simulink subsystem "AddressToWordSelector"  (R2024b)
settings: Solver=VariableStepAuto  StartTime=0.0  StopTime=10.0  RelTol=1e-3
libraries: simulink x1
settings Model: Creator=stefano  LastModifiedBy=stefano

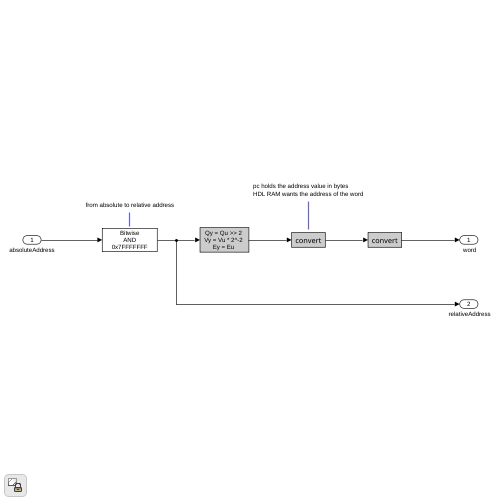
[thumbnail: Simulink's stored preview of the top-level diagram]
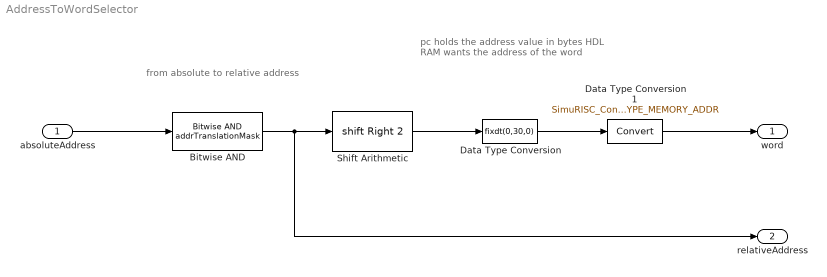
== system AddressToWordSelector ==
  note: from absolute to relative address
  note: pc holds the address value in bytes
      | HDL RAM wants the address of the word
  absoluteAddress : Inport
  Bitwise AND : simulink/Logic and Bit Operations/Bitwise Operator  logicop=AND  UseBitMask=on  BitMask=addrTranslationMask  BitMaskRealWorld=Stored Integer
      settings: LibrarySourceBlock=|
      | simulink/Quick Insert/Logic and Bit
      | Operations/Bitwise AND
  Data Type Conversion : DataTypeConversion  OutDataTypeStr=fixdt(0,30,0)  SaturateOnIntegerOverflow=off  RndMeth=Floor
  Data Type Conversion1 : DataTypeConversion  OutDataTypeStr=SimuRISC_Constants.DATATYPE_MEMORY_ADDR  SaturateOnIntegerOverflow=off  RndMeth=Floor
  Shift Arithmetic : ArithShift  BitShiftNumber=2  BitShiftDirection=Right
  " word" : Outport
  " relativeAddress" : Outport  Port=2
  wires:
  Data Type Conversion1/1 -> " word"/1
  absoluteAddress/1 -> Bitwise AND/1
  Data Type Conversion/1 -> Data Type Conversion1/1
  Bitwise AND/1 -> " relativeAddress"/1, Shift Arithmetic/1
  Shift Arithmetic/1 -> Data Type Conversion/1
